simulink subsystem "Get_Yaw_Road"  (R2022b)
settings: Solver=VariableStepAuto  StartTime=0.0  StopTime=10.0  RelTol=1e-3
settings Model: Creator=User  LastModifiedBy=User

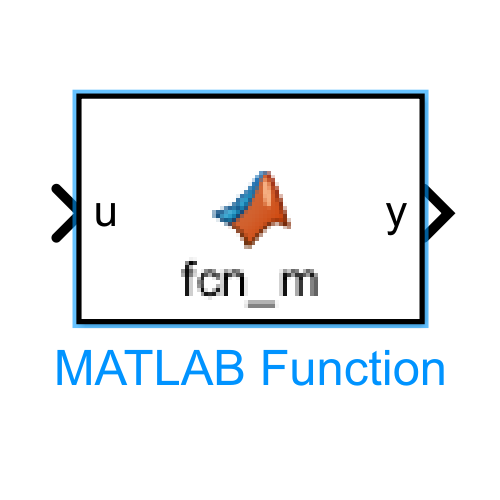
[thumbnail: Simulink's stored preview of the top-level diagram]
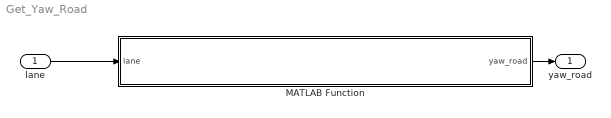
== system Get_Yaw_Road ==
  lane : Inport
  MATLAB Function : MATLAB Function  TreatAsAtomicUnit=on
  yaw_road : Outport
  wires:
  lane/1 -> MATLAB Function/1(lane)
  MATLAB Function/1(yaw_road) -> yaw_road/1

== matlab function Get_Yaw_Road/MATLAB Function ==
  data: lane input; yaw_road output
function yaw_road = get_yaw_road_m(lane)
    yaw_road = get_yaw_road(lane);
    
end
